simulink model "mpc_ObstacleAvoidance"  (R2019b)
settings: Solver=VariableStepAuto  StartTime=0.0  StopTime=5  MaxStep=1e-3  RelTol=1e-3  EnableMultiTasking=on
values from neighbouring files (symbols this model uses):
  lanes = 3    [ObstacleAvoidingUsingAdaptiveMPCExample.m]    (also in main.m; main_movingObstacle.m)
  laneWidth = 4    [ObstacleAvoidingUsingAdaptiveMPCExample.m]    (also in main.m; main_movingObstacle.m)
  obstacle = obstacleGenerateObstacleGeometryInfo(obstacle)    [ObstacleAvoidingUsingAdaptiveMPCExample.m]    (also in main.m; main_movingObstacle.m)
  u0 = [0; 0]    [ObstacleAvoidingUsingAdaptiveMPCExample.m]    (also in main.m = [0;0]; main_movingObstacle.m = [0;0])
  V = 20    [ObstacleAvoidingUsingAdaptiveMPCExample.m]    (also in main.m; main_movingObstacle.m)
  x0 = [0; 0; 0; V]    [ObstacleAvoidingUsingAdaptiveMPCExample.m]    (also in main.m = [0;0;0;V]; main_movingObstacle.m = [0;0;0;V])
libraries: mpclib x1, simulink x1
settings Model: Creator=The MathWorks, Inc.  LastModifiedBy=yeyuan
settings SolverCC: AlgebraicLoopSolver=LineSearch  MinimalZcImpactIntegration=on
settings DataIOCC: LimitDataPoints=on  SaveFormat=Array  SaveOutput=off  DSMLogging=off  SaveTime=off  ReturnWorkspaceOutputs=off
settings OptimizationCC: LifeSpan=inf
settings DebuggingCC: AlgebraicLoopMsg=none  UnderspecifiedInitializationDetection=Classic  MergeDetectMultiDrivingBlocksExec=none  SolverPrmCheckMsg=warning  AllowSymbolicDim=off  StateNameClashWarn=warning  SFUnexpectedBacktrackingDiag=warning  SFNoUnconditionalDefaultTransitionDiag=warning  SFExecutionAtInitializationDiag=none  ArithmeticOperatorsInVariantConditions=warning
settings HardwareCC: ProdBitPerPointer=32  ProdBitPerSizeT=32  ProdBitPerPtrDiffT=32  ProdLargestAtomicFloat=None  ProdIntDivRoundTo=Undefined  ProdEndianess=Unspecified  ProdWordSize=32  ProdHWDeviceType=32-bit Generic
settings ModelReferenceCC: PropagateSignalLabelsOutOfModel=off
settings SFSimCC: SimUseLocalCustomCode=off  CustomCodeUndefinedFunction=UseInterfaceOnly
settings RTWCC: RTWUseLocalCustomCode=off
settings CodeAppCC: StateflowObjectComments=on
settings GRTTargetCC: TargetLangStandard=C89/C90 (ANSI)  GeneratePreprocessorConditionals=Disable all
settings ConfigComp: CovMetricSettings=dw  CovHtmlReporting=on  CovSaveCumulativeToWorkspaceVar=on  CovSaveSingleToWorkspaceVar=on  CovExternalEMLEnable=off  CovSFcnEnable=off
settings SimscapeCC: SimscapeNormalizeSystem=off  SimscapeNominalValues="[{\"value\":\"10\",\"unit\":\"V\"},{\"value\":\"1\",\"unit\":\"A\"},{\"value\":\"10\",\"unit\":\"N*m\"},{\"value\":\"10\",\"unit\":\"bar\"},{\"value\":\"100\",\"unit\":\"kJ/kg\"},{\"value\":\"1\",\"unit\":\"kW\"},{\"value\":\"300\",\"unit\":\"K\"},{\"value\":\"100\",\"unit\":\"cm^3/s\"},{\"value\":\"1\",\"unit\":\"kN\"},{\"value\":\"1\",\"unit\":\"g/cm^3\"},{\"value\":\"1\",\"unit\":\"l\"},{\"value\":\"1\",\"unit\":\"cm^2\"},{\"value\":\"60\",\"unit\":\"Hz\"}]"
settings ConfigurationSet: Description=SimMechanics 2G
settings ExplorerConfigSet: InternalSimMechanicsExplorerSettings="<ExplorerConfiguration><canonicalview>default</canonicalview><AnimationSetting><BasePlaybackSpeed>1.0</BasePlaybackSpeed><PlaybackSpeedFactor>1.0</PlaybackSpeedFactor></AnimationSetting><TilePanel><TileInfo><Tiles Columns=\"1\" Count=\"1\" Rows=\"1\"><Column Left=\"2\" Weight=\"1\"/><Column Left=\"1552\"/><Row Top=\"2\" Weight=\"1\"/><Row Top=\"932\"/><Tile Height=\"1\" Width=\"1\" X=\"0\" Y=\"0\"/></Tiles></TileInfo><SceneInfo><SceneViewer><BGColor><R>0.60000002384185791</R><G>0.60000002384185791</G><B>0.60000002384185791</B></BGColor><Camera><Position><X>0.027865189060748197</X><Y>-2.5719092456962986</Y><Z>0.23157896538506753</Z></Position><Center><X>0.62659712312732463</X><Y>-0.46110119691712204</Y><Z>0.22087365386473376</Z></Center><Up><X>-0.0079438354874226333</X><Y>0.0073246425924307582</Y><Z>0.99994162084025784</Z></Up><Left>-0.24533778208815546</Left><Right>0.24533778208815546</Right><Bottom>-0.79734779727023208</Bottom><Top>0.79734779727023208</Top></Camera></SceneViewer></SceneInfo></TilePanel></ExplorerConfiguration>"

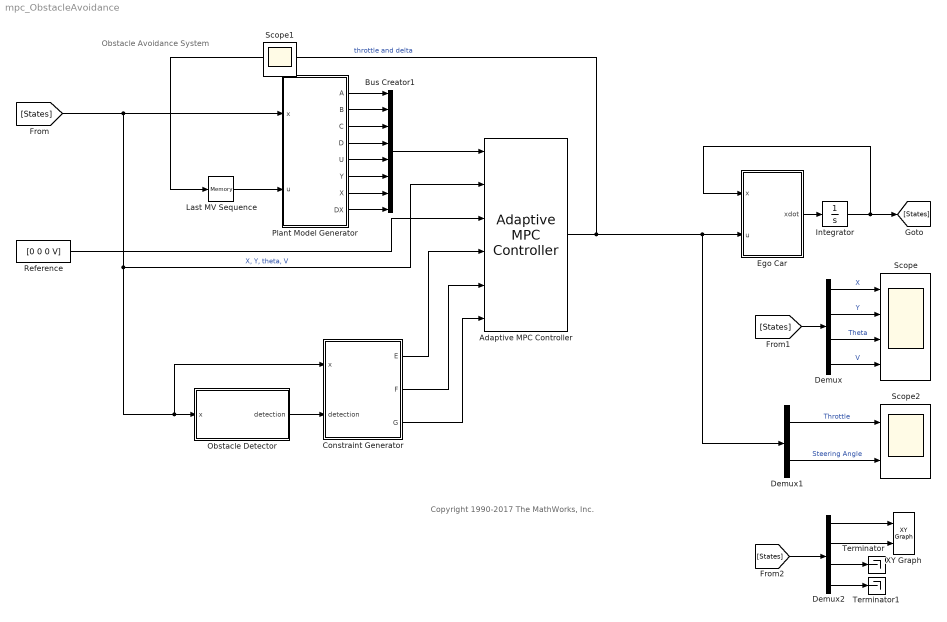
== system mpc_ObstacleAvoidance ==
  note: Obstacle Avoidance System
  note: Copyright 1990-2017 The MathWorks, Inc.
  Adaptive MPC Controller : mpclib/Adaptive MPC Controller  SCDEnableBlockLinearizationSpecification=on  mpcobj=mpcobj  enable_value=0  updateMPCinCallerWorkspace=on  md_inport=off  mv_inport=off  uref_inport=off  return_cost=off  return_mvseq=off  return_qpstatus=off  return_xseq=off  return_state=off  return_ovseq=off  state_inport=off  isltv_plant=off  umin_inport=off  umax_inport=off  ymin_inport=off  ymax_inport=off  cc_inport=on  ywt_inport=off  uwt_inport=off  duwt_inport=off  rhoeps_inport=off  pm_inport=off  MaximumP=10  HorizonChoice=FixedHorizon  BlockDataType=double  SampleTimeInherited=off  switch_inport=off
      settings: SourceProductName=Model Predictive Control Toolbox
  Bus Creator1 : BusCreator  Inputs=8
  Constraint Generator : MATLAB Function  TreatAsAtomicUnit=on
  Demux : Demux
  Demux1 : Demux  Outputs=2
  Demux2 : Demux
  Ego Car : MATLAB Function  TreatAsAtomicUnit=on
  Integrator : Integrator  InitialCondition=x0
  Last MV Sequence : Memory  InitialCondition=u0  InheritSampleTime=on
  Obstacle Detector : MATLAB Function  TreatAsAtomicUnit=on
  Plant Model Generator : MATLAB Function  TreatAsAtomicUnit=on
  Reference : Constant  Value=[0 0 0 V]
  Scope : Scope  NumInputPorts=4
  Scope2 : Scope  NumInputPorts=2
  Terminator : Terminator
  Terminator1 : Terminator
  XY Graph : simulink/Sinks/XY Graph  xmin=0  xmax=120  ymin=-6  ymax=6  st=-1
  Scope1 : Scope
  wires:
  Demux/4 -> Scope/4  "V"
  Demux/3 -> Scope/3  "Theta"
  Demux/2 -> Scope/2  "Y"
  Demux/1 -> Scope/1  "X"
  Bus Creator1/1 -> Adaptive MPC Controller/1
  Last MV Sequence/1 -> Plant Model Generator/2(u)
  Reference/1 -> Adaptive MPC Controller/3
  Plant Model Generator/1(A) -> Bus Creator1/1
  Plant Model Generator/2(B) -> Bus Creator1/2
  Plant Model Generator/3(C) -> Bus Creator1/3
  Plant Model Generator/4(D) -> Bus Creator1/4
  Plant Model Generator/5(U) -> Bus Creator1/5
  Plant Model Generator/6(Y) -> Bus Creator1/6
  Plant Model Generator/7(X) -> Bus Creator1/7
  Plant Model Generator/8(DX) -> Bus Creator1/8
  Integrator/1 -> [States], Ego Car/1(x)
  Adaptive MPC Controller/1 -> Ego Car/2(u), Demux1/1, Last MV Sequence/1  "throttle and delta"
  Ego Car/1(xdot) -> Integrator/1
  [States] -> Demux/1
  [States] -> Adaptive MPC Controller/2, Obstacle Detector/1(x), Constraint Generator/1(x), Plant Model Generator/1(x)  "X, Y, theta, V"
  Obstacle Detector/1(detection) -> Constraint Generator/2(detection)
  Constraint Generator/1(E) -> Adaptive MPC Controller/4
  Constraint Generator/2(F) -> Adaptive MPC Controller/5
  Constraint Generator/3(G) -> Adaptive MPC Controller/6
  Demux1/1 -> Scope2/1  "Throttle"
  Demux1/2 -> Scope2/2  "Steering Angle"
  [States] -> Demux2/1
  Demux2/3 -> Terminator/1
  Demux2/4 -> Terminator1/1
  Demux2/1 -> XY Graph/1
  Demux2/2 -> XY Graph/2

== matlab function mpc_ObstacleAvoidance/Ego Car ==
  settings: updateMethod=DISCRETE  sampleTime=Ts
  data: x input; u input; xdot output
function xdot = fcn(x,u)
xdot = obstacleVehicleModelCT(x,u);

== matlab function mpc_ObstacleAvoidance/Plant Model Generator ==
  settings: updateMethod=DISCRETE  sampleTime=Ts
  data: x input; u input; A output; B output; C output; D output; U output size=[2,1]; Y output size=[4,1]; X output size=[4,1]; DX output size=[4,1]; Ts parameter
function [A,B,C,D,U,Y,X,DX] = fcn(x,u,Ts)
[A,B,C,D,U,Y,X,DX] = obstacleVehicleModelDT(Ts,x,u);

== matlab function mpc_ObstacleAvoidance/Obstacle Detector ==
  settings: updateMethod=DISCRETE  sampleTime=Ts
  data: x input; obstacle parameter; laneWidth parameter; detection output
function detection  = fcn(x,obstacle,laneWidth)
% Detection Logic: it determine when the vehicle sees the obstacle
detection = obstacleDetect(x,obstacle,laneWidth);

== matlab function mpc_ObstacleAvoidance/Constraint Generator ==
  settings: updateMethod=DISCRETE  sampleTime=Ts
  data: x input; detection input; obstacle parameter; laneWidth parameter; E output; F output; G output; lanes parameter
function [E,F,G] = fcn(x,detection,obstacle,laneWidth,lanes)
% Generate run-time custom constraint
[E,F,G] = obstacleComputeCustomConstraint(x,detection,obstacle,laneWidth,lanes);
